simulink model "SIR_Temp2"  (Simulink 7.7)
settings: Solver=ode45  StartTime=0.0  StopTime=inf  MaxStep=.02  RelTol=1e-6  AbsTol=1e-4
InitFcn:
  | Initialization
values from neighbouring files (symbols this model uses):
  g = 9.81    [Initialization.m]
  lenLink1 = 0.5    [Initialization.m]
  lenLink2 = 0.5    [Initialization.m]
  mLink1 = 1    [Initialization.m]
  mLink2 = 1    [Initialization.m]
  mPin1 = 0.5    [Initialization.m]
  mPin2 = 0.5    [Initialization.m]
  rPin1 = 0.025    [Initialization.m]
libraries: mblibv1 x53, simulink x2, vrlib x1
settings Model: Creator=root  LastModifiedBy=root
settings SolverCC: AlgebraicLoopSolver=LineSearch

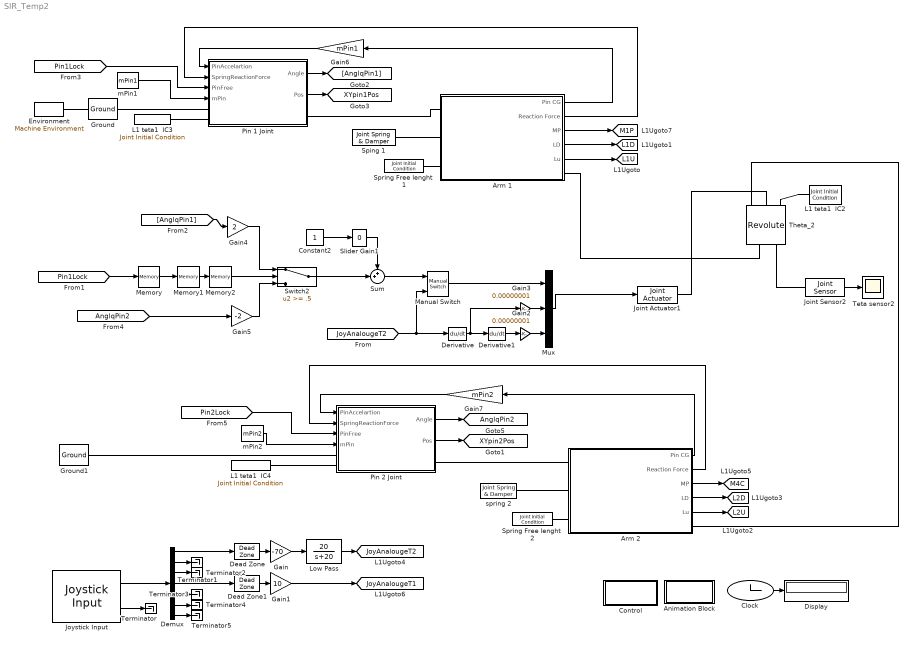
== system SIR_Temp2 ==
  Animation Block : Subsystem
  Arm 1 : Subsystem
  Arm 2 : Subsystem
  Clock : Clock
      settings: Decimation=100
  Constant2 : Constant
  Control : Subsystem
  Dead Zone : DeadZone  LowerValue=-0.1  UpperValue=0.1  SaturateOnIntegerOverflow=on
  Dead Zone1 : DeadZone  LowerValue=-0.1  UpperValue=0.1  SaturateOnIntegerOverflow=on
  Demux : Demux  Outputs=7
  Derivative : Derivative
  Derivative1 : Derivative
  Display : Display
      settings: Decimation=100
  Environment : mblibv1/Bodies/Machine Environment  SystemSampleTime=-1  PortType=env  PhysicalDomain=Mechanical  DialogTemplateClass=MECH.MachineEnvironment  SyncWhenCopied=off  Gravity=[0 -g 0]  GravityUnits=m/s^2  GravityAsSignal=off  Dimensionality=3D Only  AnalysisType=Forward dynamics  LinearAssemblyTolerance=1e-3  LinearAssemblyToleranceUnits=m  AngularAssemblyTolerance=1e-3  AngularAssemblyToleranceUnits=rad  ConstraintSolverType=Stabilizing  ConstraintRelTolerance=1e-4  ConstraintAbsTolerance=1e-4  UseRobustSingularityHandling=off  RedundancyAnalysisToleranceType=Automatically select tolerance  RedundancyAnalysisTolerance=1e-14  StatePerturbationType=Fixed  PerturbationSize=1e-5  VisualizeMachine=on  BodyVisualizationType=Use model default body geometries  BodyColorSelMode=Use model default  DefaultBodyColor=[1 0 0]
  Gain : Gain  Gain=-70
  Gain1 : Gain  Gain=10
  Gain2 : Gain  Gain=0.00000001
  Gain3 : Gain  Gain=0.00000001
  Gain4 : Gain  Gain=2
  Gain5 : Gain  Gain=-2
  Gain6 : Gain  Gain=mPin1
  Gain7 : Gain  Gain=mPin2
  Ground : mblibv1/Bodies/Ground  SystemSampleTime=-1  UpdateFromCAD=off  LeftPortType=env  RightPortType=workingframe  PhysicalDomain=Mechanical  DialogClass=GroundBlock  CoordPosition=[0 0 0]  CoordPositionUnits=m  StateVectorMgrId=1  MachineId=[2 0]  ShowEnvPort=on
  Ground1 : mblibv1/Bodies/Ground  SystemSampleTime=-1  UpdateFromCAD=off  LeftPortType=env  RightPortType=workingframe  PhysicalDomain=Mechanical  DialogClass=GroundBlock  CoordPosition=[0 0 0]  CoordPositionUnits=m  StateVectorMgrId=-1  MachineId=[0 0]  ShowEnvPort=off
  Joint Actuator1 : mblibv1/Sensors &  Actuators/Joint Actuator  SystemSampleTime=-1  UpdateFromCAD=off  PhysicalDomain=Mechanical  PortType=blob  ActuationStyle=Motion  AngleUnits=deg  ArcVelocityUnits=deg/s  ArcAccelerationUnits=deg/s^2  CoordPositionUnits=m  VelocityUnits=m/s  AccelerationUnits=m/s^2  ForceUnits=N  TorqueUnits=N*m  ActiveIO=on  Width=3  DialogClass=MechanicalActuatorBlock  Primitive=R1  ReferenceFrame=Absolute (World)
  Joint Sensor2 : mblibv1/Sensors &  Actuators/Joint Sensor  SystemSampleTime=-1  UpdateFromCAD=off  PhysicalDomain=Mechanical  PortType=blob  Muxed=off  Pose=off  Angle=off  AngleUnits=deg  ArcVelocity=off  ArcVelocityUnits=deg/s  ArcAcceleration=off  ArcAccelerationUnits=deg/s^2  CoordPosition=on  CoordPositionUnits=m  Velocity=off  VelocityUnits=m/s  Acceleration=off  AccelerationUnits=m/s^2  Quaternion=on  QuaternionDT=off  QuaternionDDT=off  QuaternionUnits=off  OutputVector=[1]  ActiveIO=on  Width=3  DialogClass=MechanicalSensorBlock  Primitive=R1  Force=off  ForceUnits=N  Torque=off  TorqueUnits=N*m  ReferenceFrame=Absolute (World)  ReactionSensedSide=Base  ReactionReferenceFrame=Absolute (World)  ReactionForce=off  ReactionForceUnits=N  ReactionMoment=on  ReactionMomentUnits=N*m
  Joystick Input : vrlib/Joystick Input  joyid=1  adjustports=on  forcefeed=off
  L1 teta1  IC2 : mblibv1/Sensors &  Actuators/Joint Initial Condition  SystemSampleTime=-1  UpdateFromCAD=off  LeftPortType=blob  RightPortType=blob  PhysicalDomain=mechanical  DialogClass=InitialConditionBlock  InitialConditions=P1$false$-0.10$m$deg$0$m/s$deg/s#P2$false$0$m$deg$2$m/s$deg/s#P3$false$0$m$deg$0$m/s$deg/s#R1$false$-50$m$deg$0$m/s$deg/s#R2$false$0$m$deg$0$m/s$deg/s#R3$false$0$m$deg$0$m/s$deg/s#S$false$0$m$deg$0$m/s$deg/s  P1PIC=0  P1VIC=0  P2PIC=0  P2VIC=0  P3PIC=0  P3VIC=0  R1PIC=0  R1VIC=0  R2PIC=0  R2VIC=0  R3PIC=0  R3VIC=0  SPIC=0  SVIC=0
  L1 teta1  IC3 : mblibv1/Sensors &  Actuators/Joint Initial Condition  SystemSampleTime=-1  UpdateFromCAD=off  LeftPortType=blob  RightPortType=blob  PhysicalDomain=mechanical  DialogClass=InitialConditionBlock  InitialConditions=P1$false$-0.10$m$deg$0$m/s$deg/s#P2$false$0$m$deg$2$m/s$deg/s#P3$false$0$m$deg$0$m/s$deg/s#R1$true$-60$m$deg$0$m/s$deg/s#R2$false$0$m$deg$0$m/s$deg/s#R3$false$0$m$deg$0$m/s$deg/s#S$false$0$m$deg$0$m/s$deg/s  P1PIC=0  P1VIC=0  P2PIC=0  P2VIC=0  P3PIC=0  P3VIC=0  R1PIC=-60  R1VIC=0  R2PIC=0  R2VIC=0  R3PIC=0  R3VIC=0  SPIC=0  SVIC=0
  L1 teta1  IC4 : mblibv1/Sensors &  Actuators/Joint Initial Condition  SystemSampleTime=-1  UpdateFromCAD=off  LeftPortType=blob  RightPortType=blob  PhysicalDomain=mechanical  DialogClass=InitialConditionBlock  InitialConditions=P1$false$-0.10$m$deg$0$m/s$deg/s#P2$false$0$m$deg$2$m/s$deg/s#P3$false$0$m$deg$0$m/s$deg/s#R1$false$-65$m$deg$0$m/s$deg/s#R2$false$0$m$deg$0$m/s$deg/s#R3$false$0$m$deg$0$m/s$deg/s#S$false$0$m$deg$0$m/s$deg/s  P1PIC=0  P1VIC=0  P2PIC=0  P2VIC=0  P3PIC=0  P3VIC=0  R1PIC=0  R1VIC=0  R2PIC=0  R2VIC=0  R3PIC=0  R3VIC=0  SPIC=0  SVIC=0
  Low Pass : TransferFcn  Numerator=[20]  Denominator=[1 20]
  Manual Switch : simulink/Signal Routing/Manual Switch  SystemSampleTime=-1  sw=1  action=0  varsize=off
  Memory : Memory
  Memory1 : Memory
  Memory2 : Memory
  Mux : Mux  Inputs=3
  Pin 1 Joint : Subsystem
  Pin 2 Joint : Subsystem
  Slider Gain1 : simulink/Math Operations/Slider Gain  SystemSampleTime=-1  low=-100  gain=0  high=100
  Sping 1 : mblibv1/Force  Elements/Joint Spring & Damper  SystemSampleTime=-1  UpdateFromCAD=off  DialogClass=JointSpringDamper  JFEParameters=P1$true$sK1$0$sFl1$m$m/s$N$deg$deg/s$N*m#P2$false$0$0$0$m$m/s$N$deg$deg/s$N*m#P3$false$0$0$0$m$m/s$N$deg$deg/s$N*m#R1$false$0$.02$0$m$m/s$N$deg$deg/s$N*m#R2$false$0$0$0$m$m/s$N$deg$deg/s$N*m#R3$false$0$0$0$m$m/s$N$deg$deg/s$N*m#S$false$0$0$0$m$m/s$N$deg$deg/s$N*m
  Spring Free lenght  1 : mblibv1/Sensors &  Actuators/Joint Initial Condition  SystemSampleTime=-1  UpdateFromCAD=off  LeftPortType=blob  RightPortType=blob  PhysicalDomain=mechanical  DialogClass=InitialConditionBlock  InitialConditions=P1$true$sFl1$m$deg$0$m/s$deg/s#P2$false$0$m$deg$2$m/s$deg/s#P3$false$0$m$deg$0$m/s$deg/s#R1$false$-65$m$deg$0$m/s$deg/s#R2$false$0$m$deg$0$m/s$deg/s#R3$false$0$m$deg$0$m/s$deg/s#S$false$0$m$deg$0$m/s$deg/s  P1PIC=sFl1  P1VIC=0  P2PIC=0  P2VIC=0  P3PIC=0  P3VIC=0  R1PIC=0  R1VIC=0  R2PIC=0  R2VIC=0  R3PIC=0  R3VIC=0  SPIC=0  SVIC=0
  Spring Free lenght  2 : mblibv1/Sensors &  Actuators/Joint Initial Condition  SystemSampleTime=-1  UpdateFromCAD=off  LeftPortType=blob  RightPortType=blob  PhysicalDomain=mechanical  DialogClass=InitialConditionBlock  InitialConditions=P1$true$sFl1$m$deg$0$m/s$deg/s#P2$false$0$m$deg$2$m/s$deg/s#P3$false$0$m$deg$0$m/s$deg/s#R1$false$-65$m$deg$0$m/s$deg/s#R2$false$0$m$deg$0$m/s$deg/s#R3$false$0$m$deg$0$m/s$deg/s#S$false$0$m$deg$0$m/s$deg/s  P1PIC=sFl1  P1VIC=0  P2PIC=0  P2VIC=0  P3PIC=0  P3VIC=0  R1PIC=0  R1VIC=0  R2PIC=0  R2VIC=0  R3PIC=0  R3VIC=0  SPIC=0  SVIC=0
  Sum : Sum  Inputs=++|
  Switch2 : Switch  Threshold=.5
  Terminator{,1..5} (6 alike) : Terminator
  Teta sensor2 : Scope
      settings: TimeRange=45  YMin=-10  YMax=10  SaveName=ScopeData6
  Theta_2 : mblibv1/Joints/Revolute  PhysicalDomain=mechanical  SubClassName=Unknown  LeftPortType=blob  RightPortType=blob  LConnTagsString=__newl0|SA1|SA2  RConnTagsString=__newr0|SA1  UpdateFromCAD=off  NumSAPorts=3  CutJoint=off  MarkAsCut=off  Primitives=prismatic  PrimitiveProps=R1$Follower$[0 0 1]$revolute  DialogClass=JointBlock  R1Axis=[0 0 1]
  mPin1 : Constant  Value=mPin1
  mPin2 : Constant  Value=mPin2
  spring 2 : mblibv1/Force  Elements/Joint Spring & Damper  SystemSampleTime=-1  UpdateFromCAD=off  DialogClass=JointSpringDamper  JFEParameters=P1$true$sK2$0$sFl2$m$m/s$N$deg$deg/s$N*m#P2$false$0$0$0$m$m/s$N$deg$deg/s$N*m#P3$false$0$0$0$m$m/s$N$deg$deg/s$N*m#R1$false$0$0$0$m$m/s$N$deg$deg/s$N*m#R2$false$0$0$0$m$m/s$N$deg$deg/s$N*m#R3$false$0$0$0$m$m/s$N$deg$deg/s$N*m#S$false$0$0$0$m$m/s$N$deg$deg/s$N*m
  tag scope: AnglqPin2=global, JoyAnalougeT1=global, JoyAnalougeT2=global, L1D=global, L1U=global, L2D=global, L2U=global, M1P=global, M4C=global, XYpin1Pos=global, XYpin2Pos=global
  wires:
  Clock/1 -> Display/1
  Joystick Input/1 -> Demux/1
  Joystick Input/2 -> Terminator/1
  Demux/3 -> Terminator2/1
  Demux/4 -> Dead Zone1/1
  Demux/5 -> Terminator3/1
  Demux/6 -> Terminator4/1
  Demux/7 -> Terminator5/1
  Dead Zone/1 -> Gain/1
  Gain/1 -> Low Pass/1
  Dead Zone1/1 -> Gain1/1
  Gain1/1 -> [JoyAnalougeT1]
  Demux/1 -> Dead Zone/1
  Demux/2 -> Terminator1/1
  Derivative/1 -> Derivative1/1, Gain3/1
  Derivative1/1 -> Gain2/1
  Low Pass/1 -> [JoyAnalougeT2]
  Joint Sensor2/1 -> Teta sensor2/1
  Gain2/1 -> Mux/3
  Gain3/1 -> Mux/2
  Arm 1/1(Pin CG) -> Gain6/1
  Gain6/1 -> Pin 1 Joint/1(PinAccelartion)
  [Pin1Lock] -> Memory/1
  mPin1/1 -> Pin 1 Joint/4(mPin)
  Pin 1 Joint/1(Angle) -> [AnglqPin1]
  Arm 1/2(Reaction Force) -> Pin 1 Joint/2(SpringReactionForce)
  Arm 1/3(MP) -> [M1P]
  Arm 1/4(LD) -> [L1D]
  Arm 1/5(Lu) -> [L1U]
  [AnglqPin1] -> Gain4/1
  Arm 2/3(MP) -> [M4C]
  Arm 2/1(Pin CG) -> Gain7/1
  mPin2/1 -> Pin 2 Joint/4(mPin)
  Constant2/1 -> Slider Gain1/1
  Slider Gain1/1 -> Sum/1
  Pin 2 Joint/1(Angle) -> [AnglqPin2]
  Pin 1 Joint/2(Pos) -> [XYpin1Pos]
  Pin 2 Joint/2(Pos) -> [XYpin2Pos]
  Memory/1 -> Memory1/1
  Memory1/1 -> Memory2/1
  Memory2/1 -> Switch2/2
  Arm 2/4(LD) -> [L2D]
  Arm 2/5(Lu) -> [L2U]
  [Pin1Lock] -> Pin 1 Joint/3(PinFree)
  Gain7/1 -> Pin 2 Joint/1(PinAccelartion)
  Arm 2/2(Reaction Force) -> Pin 2 Joint/2(SpringReactionForce)
  [Pin2Lock] -> Pin 2 Joint/3(PinFree)
  Gain4/1 -> Switch2/1
  [AnglqPin2] -> Gain5/1
  Gain5/1 -> Switch2/3
  Switch2/1 -> Sum/2
  Mux/1 -> Joint Actuator1/1
  Sum/1 -> Manual Switch/1
  Manual Switch/1 -> Mux/1
  [JoyAnalougeT2] -> Derivative/1, Manual Switch/2
  connections:
  Ground/LConn1 -- Environment/RConn1
  Joint Sensor2/LConn1 -- Theta_2/RConn2
  L1 teta1  IC2/RConn1 -- Theta_2/LConn3
  Ground/RConn1 -- Pin 1 Joint/LConn1
  Joint Actuator1/RConn1 -- Theta_2/LConn2
  Pin 1 Joint/RConn1 -- Arm 1/LConn1
  L1 teta1  IC3/RConn1 -- Pin 1 Joint/LConn2
  Sping 1/LConn1 -- Arm 1/LConn2
  Spring Free lenght  1/RConn1 -- Arm 1/LConn3
  spring 2/LConn1 -- Arm 2/LConn2
  Arm 2/LConn3 -- Spring Free lenght  2/RConn1
  Pin 2 Joint/LConn1 -- Ground1/RConn1
  L1 teta1  IC4/RConn1 -- Pin 2 Joint/LConn2
  Arm 2/LConn1 -- Pin 2 Joint/RConn1
  Theta_2/RConn1 -- Arm 1/RConn1
  Theta_2/LConn1 -- Arm 2/RConn1

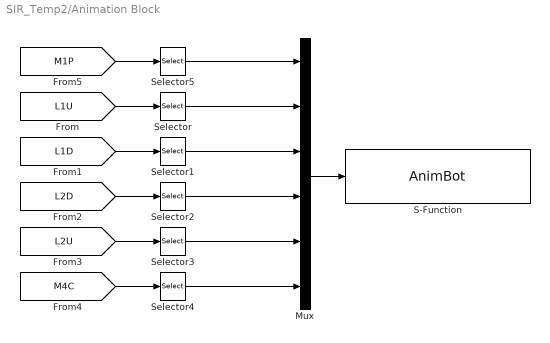
== system SIR_Temp2/Animation Block ==
  Mux : Mux  Inputs=6
  S-Function : S-Function  FunctionName=AnimBot  Parameters=0.001  EnableBusSupport=off
  Selector{,1..5} (6 alike) : Selector  InputPortWidth=3  IndexOptions=Index vector (dialog)  Indices=[1 2]  OutputSizes=1
  wires:
  Mux/1 -> S-Function/1
  [M4C] -> Selector4/1
  [L2U] -> Selector3/1
  [L2D] -> Selector2/1
  [L1D] -> Selector1/1
  [L1U] -> Selector/1
  [M1P] -> Selector5/1
  Selector5/1 -> Mux/1
  Selector/1 -> Mux/2
  Selector1/1 -> Mux/3
  Selector2/1 -> Mux/4
  Selector3/1 -> Mux/5
  Selector4/1 -> Mux/6

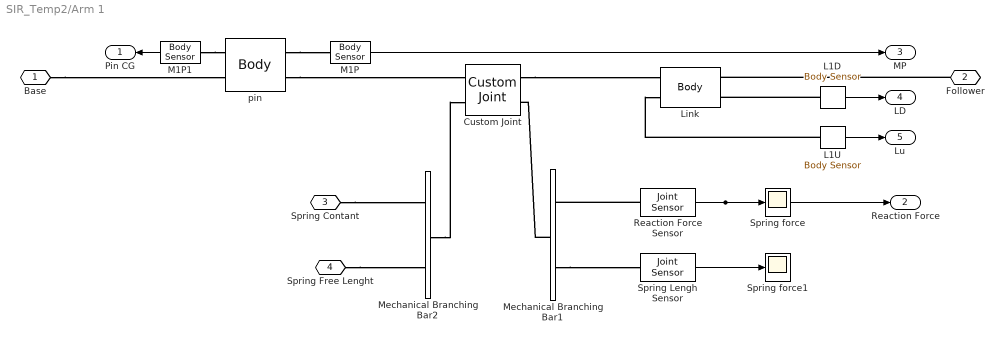
== system SIR_Temp2/Arm 1 ==
  Custom Joint : mblibv1/Joints/Custom Joint  PhysicalDomain=mechanical  SubClassName=custom_joint  LeftPortType=blob  RightPortType=blob  LConnTagsString=__newl0|SA1  RConnTagsString=__newr0|SA1  UpdateFromCAD=off  NumSAPorts=2  CutJoint=off  MarkAsCut=off  Primitives=prismatic  PrimitiveProps=P1$World$[0 1 0]$Prismatic  DialogClass=JointBlock  R1Axis=[]  R2Axis=[]  R3Axis=[]  P1Axis=[0 1 0]  P2Axis=[]  P3Axis=[]  SAxis=[]
  L1D : mblibv1/Sensors &  Actuators/Body Sensor  SystemSampleTime=-1  UpdateFromCAD=off  PhysicalDomain=Mechanical  PortType=blob  Muxed=on  Pose=off  Angle=on  AngleUnits=deg  ArcVelocity=off  ArcVelocityUnits=deg/s  ArcAcceleration=off  ArcAccelerationUnits=deg/s^2  CoordPosition=on  CoordPositionUnits=m  Velocity=off  VelocityUnits=m/s  Acceleration=off  AccelerationUnits=m/s^2  Quaternion=on  QuaternionDT=off  QuaternionDDT=off  QuaternionUnits=off  OutputVector=[1]  ActiveIO=on  Width=3  DialogClass=MechanicalSensorBlock  ReferenceFrame=Absolute (World)
  L1U : mblibv1/Sensors &  Actuators/Body Sensor  SystemSampleTime=-1  UpdateFromCAD=off  PhysicalDomain=Mechanical  PortType=blob  Muxed=on  Pose=off  Angle=on  AngleUnits=deg  ArcVelocity=off  ArcVelocityUnits=deg/s  ArcAcceleration=off  ArcAccelerationUnits=deg/s^2  CoordPosition=on  CoordPositionUnits=m  Velocity=off  VelocityUnits=m/s  Acceleration=off  AccelerationUnits=m/s^2  Quaternion=on  QuaternionDT=off  QuaternionDDT=off  QuaternionUnits=off  OutputVector=[1]  ActiveIO=on  Width=3  DialogClass=MechanicalSensorBlock  ReferenceFrame=Absolute (World)
  Link : mblibv1/Bodies/Body  PhysicalDomain=mechanical  SubClassName=Unknown  LeftPortType=workingframe  RightPortType=workingframe  LConnTagsString=CS1|CS3  RConnTagsString=CS2|CS4  UpdateFromCAD=off  DialogClass=MechanicalBodyBlock  Mass=mLink1  MassUnits=kg  InertiaUnits=kg*m^2  Inertia=mLink1/12*[lenLink1 0 0; 0 0 0; 0 0 lenLink1]  Shape=Cylinder  ShapeDims=[1 1]  ShapeUnits=m  ShapeUse=false  Density=1  DensityUnits=kg/m^3  DensityUse=false  GraphicsMode=MACHINE_DEFAULT  BodyColorSelMode=MACHINE_DEFAULT  BodyColor=[1 0 0]  AttachedToCS=CG  CG=Left$CG$[0 -0.25 0]$CS1$CS1$m$[0 0 0]$Euler X-Y-Z$deg$WORLD$false$none  WorkingFrames=Left$CS1$[0 0 0]$Adjoining$Adjoining$m$[0 0 0]$Euler X-Y-Z$deg$WORLD$true$none#Left$CS3$[0 0 0]$CS1$CS1$m$[0 0 0]$Euler X-Y-Z$deg$WORLD$true$none#Right$CS2$[0 -0.5 0]$CS1$CS1$m$[0 0 0]$Euler X-Y-Z$deg$WORLD$true$none#Right$CS4$[0 -0.5 0]$CS1$CS1$m$[0 0 0]$Euler X-Y-Z$deg$WORLD$true$none  CGPos=[0 -0.25 0]  CGRot=[0 0 0]  CS0Pos=[]  CS0Rot=[]  CS1Pos=[0 0 0]  CS1Rot=[0 0 0]  CS2Pos=[0 -0.5 0]  CS2Rot=[0 0 0]  CS3Pos=[0 0 0]  CS3Rot=[0 0 0]  CS4Pos=[0 -0.5 0]  CS4Rot=[0 0 0]  CS5Pos=[]  CS5Rot=[]  CS6Pos=[]  CS6Rot=[]  CS7Pos=[]  CS7Rot=[]  CS8Pos=[]  CS8Rot=[]  CS9Pos=[]  CS9Rot=[]  CS10Pos=[]  CS10Rot=[]  CS11Pos=[]  CS11Rot=[]  CS12Pos=[]  CS12Rot=[]  CS13Pos=[]  CS13Rot=[]  CS14Pos=[]  CS14Rot=[]  CS15Pos=[]  CS15Rot=[]  CS16Pos=[]  CS16Rot=[]  CS17Pos=[]  CS17Rot=[]  CS18Pos=[]  CS18Rot=[]  CS19Pos=[]  CS19Rot=[]  CS20Pos=[]  CS20Rot=[]
  M1P : mblibv1/Sensors &  Actuators/Body Sensor  SystemSampleTime=-1  UpdateFromCAD=off  PhysicalDomain=Mechanical  PortType=blob  Muxed=on  Pose=off  Angle=on  AngleUnits=deg  ArcVelocity=off  ArcVelocityUnits=deg/s  ArcAcceleration=off  ArcAccelerationUnits=deg/s^2  CoordPosition=on  CoordPositionUnits=m  Velocity=off  VelocityUnits=m/s  Acceleration=off  AccelerationUnits=m/s^2  Quaternion=on  QuaternionDT=off  QuaternionDDT=off  QuaternionUnits=off  OutputVector=[1]  ActiveIO=on  Width=3  DialogClass=MechanicalSensorBlock  ReferenceFrame=Absolute (World)
  M1P1 : mblibv1/Sensors &  Actuators/Body Sensor  SystemSampleTime=-1  UpdateFromCAD=off  PhysicalDomain=Mechanical  PortType=blob  Muxed=on  Pose=off  Angle=on  AngleUnits=deg  ArcVelocity=off  ArcVelocityUnits=deg/s  ArcAcceleration=off  ArcAccelerationUnits=deg/s^2  CoordPosition=off  CoordPositionUnits=m  Velocity=off  VelocityUnits=m/s  Acceleration=on  AccelerationUnits=m/s^2  Quaternion=on  QuaternionDT=off  QuaternionDDT=off  QuaternionUnits=off  OutputVector=[1]  ActiveIO=on  Width=3  DialogClass=MechanicalSensorBlock  ReferenceFrame=Absolute (World)
  Mechanical Branching Bar1 : mblibv1/Utilities/Mechanical Branching Bar  PhysicalDomain=mechanical  SubClassName=Unknown  LeftPortType=blob  RightPortType=blob  LConnTagsString=_newl0  RConnTagsString=__newr0|SA2  UpdateFromCAD=off  DialogClass=MechanicalBranchingBarBlock  NumSAPorts=2
  Mechanical Branching Bar2 : mblibv1/Utilities/Mechanical Branching Bar  PhysicalDomain=mechanical  SubClassName=Unknown  LeftPortType=blob  RightPortType=blob  LConnTagsString=_newl0  RConnTagsString=__newr0|SA2  UpdateFromCAD=off  DialogClass=MechanicalBranchingBarBlock  NumSAPorts=2
  "Reaction Force Sensor " : mblibv1/Sensors &  Actuators/Joint Sensor  SystemSampleTime=-1  UpdateFromCAD=off  PhysicalDomain=Mechanical  PortType=blob  Muxed=off  Pose=off  Angle=on  AngleUnits=deg  ArcVelocity=off  ArcVelocityUnits=deg/s  ArcAcceleration=off  ArcAccelerationUnits=deg/s^2  CoordPosition=off  CoordPositionUnits=m  Velocity=off  VelocityUnits=m/s  Acceleration=off  AccelerationUnits=m/s^2  Quaternion=on  QuaternionDT=off  QuaternionDDT=off  QuaternionUnits=off  OutputVector=[1]  ActiveIO=on  Width=3  DialogClass=MechanicalSensorBlock  Primitive=P1  Force=off  ForceUnits=N  Torque=off  TorqueUnits=N*m  ReferenceFrame=Absolute (World)  ReactionSensedSide=Base  ReactionReferenceFrame=Absolute (World)  ReactionForce=on  ReactionForceUnits=N  ReactionMoment=off  ReactionMomentUnits=N*m
  Spring Lengh Sensor : mblibv1/Sensors &  Actuators/Joint Sensor  SystemSampleTime=-1  UpdateFromCAD=off  PhysicalDomain=Mechanical  PortType=blob  Muxed=off  Pose=off  Angle=on  AngleUnits=deg  ArcVelocity=off  ArcVelocityUnits=deg/s  ArcAcceleration=off  ArcAccelerationUnits=deg/s^2  CoordPosition=off  CoordPositionUnits=m  Velocity=off  VelocityUnits=m/s  Acceleration=off  AccelerationUnits=m/s^2  Quaternion=on  QuaternionDT=off  QuaternionDDT=off  QuaternionUnits=off  OutputVector=[1]  ActiveIO=on  Width=3  DialogClass=MechanicalSensorBlock  Primitive=P1  Force=off  ForceUnits=N  Torque=off  TorqueUnits=N*m  ReferenceFrame=Absolute (World)  ReactionSensedSide=Base  ReactionReferenceFrame=Absolute (World)  ReactionForce=on  ReactionForceUnits=N  ReactionMoment=off  ReactionMomentUnits=N*m
  Spring force : Scope
      settings: TimeRange=0.45  YMin=-10  YMax=1  SaveName=ScopeData22
  Spring force1 : Scope
      settings: TimeRange=0.45  YMin=-10  YMax=1  SaveName=ScopeData8
  pin : mblibv1/Bodies/Body  PhysicalDomain=mechanical  SubClassName=Unknown  LeftPortType=workingframe  RightPortType=workingframe  LConnTagsString=CG|CS3  RConnTagsString=CS2|CS4  UpdateFromCAD=off  DialogClass=MechanicalBodyBlock  Mass=mPin1  MassUnits=kg  InertiaUnits=kg*m^2  Inertia=2/5*mPin1*(rPin1)^2*[1 0 0; 0 1 0; 0 0 1]  Shape=Cylinder  ShapeDims=[1 1]  ShapeUnits=m  ShapeUse=false  Density=1  DensityUnits=kg/m^3  DensityUse=false  GraphicsMode=MACHINE_DEFAULT  BodyColorSelMode=MACHINE_DEFAULT  BodyColor=[1 0 0]  AttachedToCS=CG  CG=Left$CG$[0 -0.025 0]$CS3$CS3$m$[0 0 0]$Euler X-Y-Z$deg$WORLD$true$none  WorkingFrames=Left$CS3$[0 0 0]$Adjoining$Adjoining$m$[0 0 0]$Euler X-Y-Z$deg$WORLD$true$none#Right$CS2$[0 -.025 0]$CS3$CS3$m$[0 0 0]$Euler X-Y-Z$deg$WORLD$true$none#Right$CS4$[0 -.05 0]$CS3$CS3$m$[0 0 0]$Euler X-Y-Z$deg$WORLD$true$none  CGPos=[0 -0.025 0]  CGRot=[0 0 0]  CS0Pos=[]  CS0Rot=[]  CS1Pos=[]  CS1Rot=[]  CS2Pos=[0 -.025 0]  CS2Rot=[0 0 0]  CS3Pos=[0 0 0]  CS3Rot=[0 0 0]  CS4Pos=[0 -.05 0]  CS4Rot=[0 0 0]  CS5Pos=[]  CS5Rot=[]  CS6Pos=[]  CS6Rot=[]  CS7Pos=[]  CS7Rot=[]  CS8Pos=[]  CS8Rot=[]  CS9Pos=[]  CS9Rot=[]  CS10Pos=[]  CS10Rot=[]  CS11Pos=[]  CS11Rot=[]  CS12Pos=[]  CS12Rot=[]  CS13Pos=[]  CS13Rot=[]  CS14Pos=[]  CS14Rot=[]  CS15Pos=[]  CS15Rot=[]  CS16Pos=[]  CS16Rot=[]  CS17Pos=[]  CS17Rot=[]  CS18Pos=[]  CS18Rot=[]  CS19Pos=[]  CS19Rot=[]  CS20Pos=[]  CS20Rot=[]
  Base : PMIOPort  Port=1  Side=Left
  Follower : PMIOPort  Port=2  Side=Right
  Spring Contant : PMIOPort  Port=3  Side=Left
  Spring Free Lenght : PMIOPort  Port=4  Side=Left
  Pin CG : Outport
  Reaction Force : Outport  Port=2
  MP : Outport  Port=3
  LD : Outport  Port=4
  Lu : Outport  Port=5
  wires:
  L1U/1 -> Lu/1
  L1D/1 -> LD/1
  M1P1/1 -> Pin CG/1
  "Reaction Force Sensor "/1 -> Reaction Force/1, Spring force/1
  Spring Lengh Sensor/1 -> Spring force1/1
  M1P/1 -> MP/1
  connections:
  pin/RConn2 -- Custom Joint/LConn1
  Mechanical Branching Bar2/LConn1 -- Custom Joint/LConn2
  Mechanical Branching Bar1/LConn1 -- Custom Joint/RConn2
  L1D/LConn1 -- Link/RConn2
  L1U/LConn1 -- Link/LConn2
  pin/RConn1 -- M1P/LConn1
  M1P1/LConn1 -- pin/LConn1
  "Reaction Force Sensor "/LConn1 -- Mechanical Branching Bar1/RConn1
  Base/RConn1 -- pin/LConn2
  Follower/RConn1 -- Link/RConn1
  Custom Joint/RConn1 -- Link/LConn1
  Mechanical Branching Bar1/RConn2 -- Spring Lengh Sensor/LConn1
  Spring Contant/RConn1 -- Mechanical Branching Bar2/RConn1
  Spring Free Lenght/RConn1 -- Mechanical Branching Bar2/RConn2

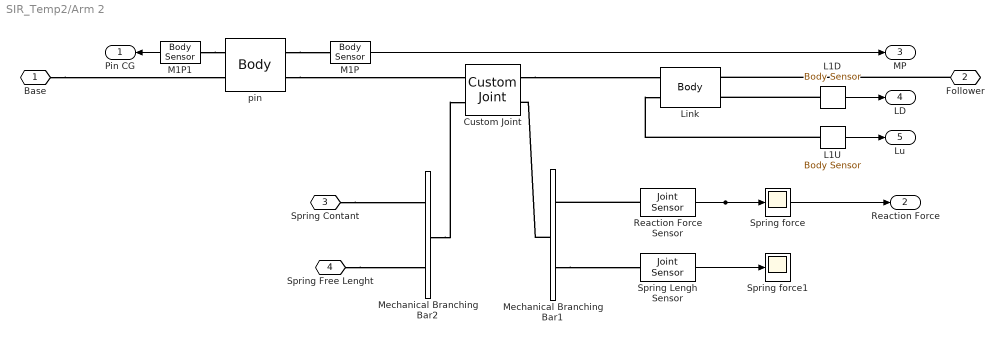
== system SIR_Temp2/Arm 2 ==
  Custom Joint : mblibv1/Joints/Custom Joint  PhysicalDomain=mechanical  SubClassName=custom_joint  LeftPortType=blob  RightPortType=blob  LConnTagsString=__newl0|SA1  RConnTagsString=__newr0|SA1  UpdateFromCAD=off  NumSAPorts=2  CutJoint=off  MarkAsCut=off  Primitives=prismatic  PrimitiveProps=P1$World$[0 1 0]$Prismatic  DialogClass=JointBlock  R1Axis=[]  R2Axis=[]  R3Axis=[]  P1Axis=[0 1 0]  P2Axis=[]  P3Axis=[]  SAxis=[]
  L1D : mblibv1/Sensors &  Actuators/Body Sensor  SystemSampleTime=-1  UpdateFromCAD=off  PhysicalDomain=Mechanical  PortType=blob  Muxed=on  Pose=off  Angle=on  AngleUnits=deg  ArcVelocity=off  ArcVelocityUnits=deg/s  ArcAcceleration=off  ArcAccelerationUnits=deg/s^2  CoordPosition=on  CoordPositionUnits=m  Velocity=off  VelocityUnits=m/s  Acceleration=off  AccelerationUnits=m/s^2  Quaternion=on  QuaternionDT=off  QuaternionDDT=off  QuaternionUnits=off  OutputVector=[1]  ActiveIO=on  Width=3  DialogClass=MechanicalSensorBlock  ReferenceFrame=Absolute (World)
  L1U : mblibv1/Sensors &  Actuators/Body Sensor  SystemSampleTime=-1  UpdateFromCAD=off  PhysicalDomain=Mechanical  PortType=blob  Muxed=on  Pose=off  Angle=on  AngleUnits=deg  ArcVelocity=off  ArcVelocityUnits=deg/s  ArcAcceleration=off  ArcAccelerationUnits=deg/s^2  CoordPosition=on  CoordPositionUnits=m  Velocity=off  VelocityUnits=m/s  Acceleration=off  AccelerationUnits=m/s^2  Quaternion=on  QuaternionDT=off  QuaternionDDT=off  QuaternionUnits=off  OutputVector=[1]  ActiveIO=on  Width=3  DialogClass=MechanicalSensorBlock  ReferenceFrame=Absolute (World)
  Link : mblibv1/Bodies/Body  PhysicalDomain=mechanical  SubClassName=Unknown  LeftPortType=workingframe  RightPortType=workingframe  LConnTagsString=CS1|CS3  RConnTagsString=CS2|CS4  UpdateFromCAD=off  DialogClass=MechanicalBodyBlock  Mass=mLink2  MassUnits=kg  InertiaUnits=kg*m^2  Inertia=mLink2/12*[lenLink2 0 0; 0 0 0; 0 0 lenLink2]  Shape=Cylinder  ShapeDims=[1 1]  ShapeUnits=m  ShapeUse=false  Density=1  DensityUnits=kg/m^3  DensityUse=false  GraphicsMode=MACHINE_DEFAULT  BodyColorSelMode=MACHINE_DEFAULT  BodyColor=[1 0 0]  AttachedToCS=CG  CG=Left$CG$[0 -0.25 0]$CS1$CS1$m$[0 0 0]$Euler X-Y-Z$deg$WORLD$false$none  WorkingFrames=Left$CS1$[0 0 0]$Adjoining$Adjoining$m$[0 0 0]$Euler X-Y-Z$deg$WORLD$true$none#Left$CS3$[0 0 0]$CS1$CS1$m$[0 0 0]$Euler X-Y-Z$deg$WORLD$true$none#Right$CS2$[0 -0.5 0]$CS1$CS1$m$[0 0 0]$Euler X-Y-Z$deg$WORLD$true$none#Right$CS4$[0 -0.5 0]$CS1$CS1$m$[0 0 0]$Euler X-Y-Z$deg$WORLD$true$none  CGPos=[0 -0.25 0]  CGRot=[0 0 0]  CS0Pos=[]  CS0Rot=[]  CS1Pos=[0 0 0]  CS1Rot=[0 0 0]  CS2Pos=[0 -0.5 0]  CS2Rot=[0 0 0]  CS3Pos=[0 0 0]  CS3Rot=[0 0 0]  CS4Pos=[0 -0.5 0]  CS4Rot=[0 0 0]  CS5Pos=[]  CS5Rot=[]  CS6Pos=[]  CS6Rot=[]  CS7Pos=[]  CS7Rot=[]  CS8Pos=[]  CS8Rot=[]  CS9Pos=[]  CS9Rot=[]  CS10Pos=[]  CS10Rot=[]  CS11Pos=[]  CS11Rot=[]  CS12Pos=[]  CS12Rot=[]  CS13Pos=[]  CS13Rot=[]  CS14Pos=[]  CS14Rot=[]  CS15Pos=[]  CS15Rot=[]  CS16Pos=[]  CS16Rot=[]  CS17Pos=[]  CS17Rot=[]  CS18Pos=[]  CS18Rot=[]  CS19Pos=[]  CS19Rot=[]  CS20Pos=[]  CS20Rot=[]
  M1P : mblibv1/Sensors &  Actuators/Body Sensor  SystemSampleTime=-1  UpdateFromCAD=off  PhysicalDomain=Mechanical  PortType=blob  Muxed=on  Pose=off  Angle=on  AngleUnits=deg  ArcVelocity=off  ArcVelocityUnits=deg/s  ArcAcceleration=off  ArcAccelerationUnits=deg/s^2  CoordPosition=on  CoordPositionUnits=m  Velocity=off  VelocityUnits=m/s  Acceleration=off  AccelerationUnits=m/s^2  Quaternion=on  QuaternionDT=off  QuaternionDDT=off  QuaternionUnits=off  OutputVector=[1]  ActiveIO=on  Width=3  DialogClass=MechanicalSensorBlock  ReferenceFrame=Absolute (World)
  M1P1 : mblibv1/Sensors &  Actuators/Body Sensor  SystemSampleTime=-1  UpdateFromCAD=off  PhysicalDomain=Mechanical  PortType=blob  Muxed=on  Pose=off  Angle=on  AngleUnits=deg  ArcVelocity=off  ArcVelocityUnits=deg/s  ArcAcceleration=off  ArcAccelerationUnits=deg/s^2  CoordPosition=off  CoordPositionUnits=m  Velocity=off  VelocityUnits=m/s  Acceleration=on  AccelerationUnits=m/s^2  Quaternion=on  QuaternionDT=off  QuaternionDDT=off  QuaternionUnits=off  OutputVector=[1]  ActiveIO=on  Width=3  DialogClass=MechanicalSensorBlock  ReferenceFrame=Absolute (World)
  Mechanical Branching Bar1 : mblibv1/Utilities/Mechanical Branching Bar  PhysicalDomain=mechanical  SubClassName=Unknown  LeftPortType=blob  RightPortType=blob  LConnTagsString=_newl0  RConnTagsString=__newr0|SA2  UpdateFromCAD=off  DialogClass=MechanicalBranchingBarBlock  NumSAPorts=2
  Mechanical Branching Bar2 : mblibv1/Utilities/Mechanical Branching Bar  PhysicalDomain=mechanical  SubClassName=Unknown  LeftPortType=blob  RightPortType=blob  LConnTagsString=_newl0  RConnTagsString=__newr0|SA2  UpdateFromCAD=off  DialogClass=MechanicalBranchingBarBlock  NumSAPorts=2
  "Reaction Force Sensor " : mblibv1/Sensors &  Actuators/Joint Sensor  SystemSampleTime=-1  UpdateFromCAD=off  PhysicalDomain=Mechanical  PortType=blob  Muxed=off  Pose=off  Angle=on  AngleUnits=deg  ArcVelocity=off  ArcVelocityUnits=deg/s  ArcAcceleration=off  ArcAccelerationUnits=deg/s^2  CoordPosition=off  CoordPositionUnits=m  Velocity=off  VelocityUnits=m/s  Acceleration=off  AccelerationUnits=m/s^2  Quaternion=on  QuaternionDT=off  QuaternionDDT=off  QuaternionUnits=off  OutputVector=[1]  ActiveIO=on  Width=3  DialogClass=MechanicalSensorBlock  Primitive=P1  Force=off  ForceUnits=N  Torque=off  TorqueUnits=N*m  ReferenceFrame=Absolute (World)  ReactionSensedSide=Base  ReactionReferenceFrame=Absolute (World)  ReactionForce=on  ReactionForceUnits=N  ReactionMoment=off  ReactionMomentUnits=N*m
  Spring Lengh Sensor : mblibv1/Sensors &  Actuators/Joint Sensor  SystemSampleTime=-1  UpdateFromCAD=off  PhysicalDomain=Mechanical  PortType=blob  Muxed=off  Pose=off  Angle=on  AngleUnits=deg  ArcVelocity=off  ArcVelocityUnits=deg/s  ArcAcceleration=off  ArcAccelerationUnits=deg/s^2  CoordPosition=off  CoordPositionUnits=m  Velocity=off  VelocityUnits=m/s  Acceleration=off  AccelerationUnits=m/s^2  Quaternion=on  QuaternionDT=off  QuaternionDDT=off  QuaternionUnits=off  OutputVector=[1]  ActiveIO=on  Width=3  DialogClass=MechanicalSensorBlock  Primitive=P1  Force=off  ForceUnits=N  Torque=off  TorqueUnits=N*m  ReferenceFrame=Absolute (World)  ReactionSensedSide=Base  ReactionReferenceFrame=Absolute (World)  ReactionForce=on  ReactionForceUnits=N  ReactionMoment=off  ReactionMomentUnits=N*m
  Spring force : Scope
      settings: TimeRange=0.45  YMin=-10  YMax=1  SaveName=ScopeData22
  Spring force1 : Scope
      settings: TimeRange=0.45  YMin=-10  YMax=1  SaveName=ScopeData8
  pin : mblibv1/Bodies/Body  PhysicalDomain=mechanical  SubClassName=Unknown  LeftPortType=workingframe  RightPortType=workingframe  LConnTagsString=CG|CS3  RConnTagsString=CS2|CS4  UpdateFromCAD=off  DialogClass=MechanicalBodyBlock  Mass=mPin1  MassUnits=kg  InertiaUnits=kg*m^2  Inertia=2/5*mPin1*(rPin1)^2*[1 0 0; 0 1 0; 0 0 1]  Shape=Cylinder  ShapeDims=[1 1]  ShapeUnits=m  ShapeUse=false  Density=1  DensityUnits=kg/m^3  DensityUse=false  GraphicsMode=MACHINE_DEFAULT  BodyColorSelMode=MACHINE_DEFAULT  BodyColor=[1 0 0]  AttachedToCS=CG  CG=Left$CG$[0 -0.025 0]$CS3$CS3$m$[0 0 0]$Euler X-Y-Z$deg$WORLD$true$none  WorkingFrames=Left$CS3$[0 0 0]$Adjoining$Adjoining$m$[0 0 0]$Euler X-Y-Z$deg$WORLD$true$none#Right$CS2$[0 -.025 0]$CS3$CS3$m$[0 0 0]$Euler X-Y-Z$deg$WORLD$true$none#Right$CS4$[0 -.05 0]$CS3$CS3$m$[0 0 0]$Euler X-Y-Z$deg$WORLD$true$none  CGPos=[0 -0.025 0]  CGRot=[0 0 0]  CS0Pos=[]  CS0Rot=[]  CS1Pos=[]  CS1Rot=[]  CS2Pos=[0 -.025 0]  CS2Rot=[0 0 0]  CS3Pos=[0 0 0]  CS3Rot=[0 0 0]  CS4Pos=[0 -.05 0]  CS4Rot=[0 0 0]  CS5Pos=[]  CS5Rot=[]  CS6Pos=[]  CS6Rot=[]  CS7Pos=[]  CS7Rot=[]  CS8Pos=[]  CS8Rot=[]  CS9Pos=[]  CS9Rot=[]  CS10Pos=[]  CS10Rot=[]  CS11Pos=[]  CS11Rot=[]  CS12Pos=[]  CS12Rot=[]  CS13Pos=[]  CS13Rot=[]  CS14Pos=[]  CS14Rot=[]  CS15Pos=[]  CS15Rot=[]  CS16Pos=[]  CS16Rot=[]  CS17Pos=[]  CS17Rot=[]  CS18Pos=[]  CS18Rot=[]  CS19Pos=[]  CS19Rot=[]  CS20Pos=[]  CS20Rot=[]
  Base : PMIOPort  Port=1  Side=Left
  Follower : PMIOPort  Port=2  Side=Right
  Spring Contant : PMIOPort  Port=3  Side=Left
  Spring Free Lenght : PMIOPort  Port=4  Side=Left
  Pin CG : Outport
  Reaction Force : Outport  Port=2
  MP : Outport  Port=3
  LD : Outport  Port=4
  Lu : Outport  Port=5
  wires:
  L1U/1 -> Lu/1
  L1D/1 -> LD/1
  M1P1/1 -> Pin CG/1
  "Reaction Force Sensor "/1 -> Reaction Force/1, Spring force/1
  Spring Lengh Sensor/1 -> Spring force1/1
  M1P/1 -> MP/1
  connections:
  pin/RConn2 -- Custom Joint/LConn1
  Mechanical Branching Bar2/LConn1 -- Custom Joint/LConn2
  Mechanical Branching Bar1/LConn1 -- Custom Joint/RConn2
  L1D/LConn1 -- Link/RConn2
  L1U/LConn1 -- Link/LConn2
  pin/RConn1 -- M1P/LConn1
  M1P1/LConn1 -- pin/LConn1
  "Reaction Force Sensor "/LConn1 -- Mechanical Branching Bar1/RConn1
  Base/RConn1 -- pin/LConn2
  Follower/RConn1 -- Link/RConn1
  Custom Joint/RConn1 -- Link/LConn1
  Mechanical Branching Bar1/RConn2 -- Spring Lengh Sensor/LConn1
  Spring Contant/RConn1 -- Mechanical Branching Bar2/RConn1
  Spring Free Lenght/RConn1 -- Mechanical Branching Bar2/RConn2

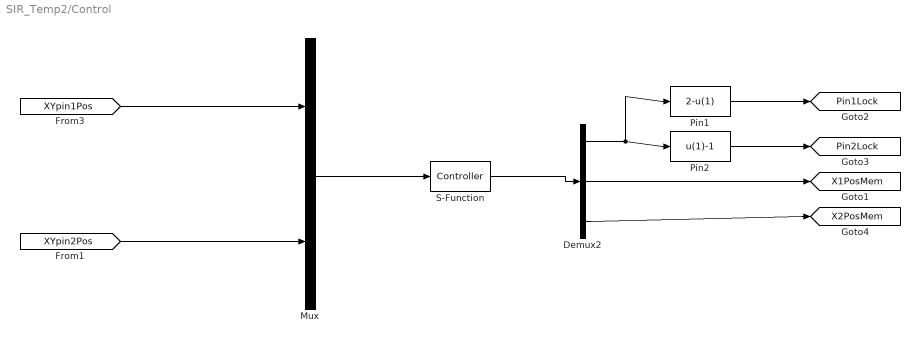
== system SIR_Temp2/Control ==
  Demux2 : Demux  Outputs=3
  Mux : Mux  Inputs=2
  Pin1 : Fcn  Expr=2-u(1)
  Pin2 : Fcn  Expr=u(1)-1
  S-Function : S-Function  FunctionName=Controller  Parameters=0.001  EnableBusSupport=off
  tag scope: Pin1Lock=global, Pin2Lock=global, X1PosMem=global, X2PosMem=global
  wires:
  Mux/1 -> S-Function/1
  Pin1/1 -> [Pin1Lock]
  Pin2/1 -> [Pin2Lock]
  [XYpin1Pos] -> Mux/1
  [XYpin2Pos] -> Mux/2
  S-Function/1 -> Demux2/1
  Demux2/1 -> Pin1/1, Pin2/1
  Demux2/2 -> [X1PosMem]
  Demux2/3 -> [X2PosMem]

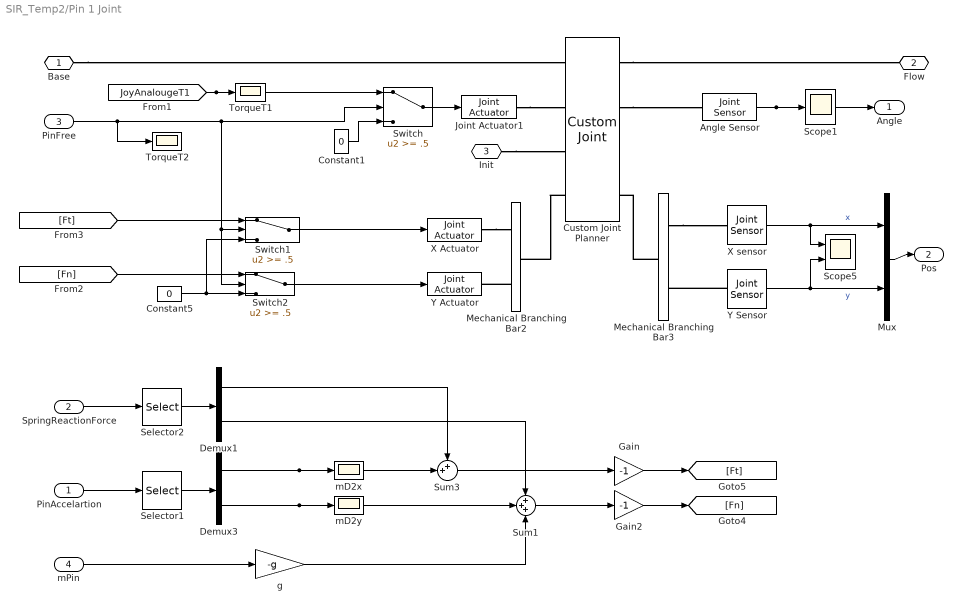
== system SIR_Temp2/Pin 1 Joint ==
  PinAccelartion : Inport
  SpringReactionForce : Inport  Port=2
  PinFree : Inport  Port=3
  mPin : Inport  Port=4
  Angle Sensor : mblibv1/Sensors &  Actuators/Joint Sensor  SystemSampleTime=-1  UpdateFromCAD=off  PhysicalDomain=Mechanical  PortType=blob  Muxed=off  Pose=off  Angle=on  AngleUnits=deg  ArcVelocity=off  ArcVelocityUnits=deg/s  ArcAcceleration=off  ArcAccelerationUnits=deg/s^2  CoordPosition=on  CoordPositionUnits=m  Velocity=off  VelocityUnits=m/s  Acceleration=off  AccelerationUnits=m/s^2  Quaternion=on  QuaternionDT=off  QuaternionDDT=off  QuaternionUnits=off  OutputVector=[1]  ActiveIO=on  Width=1  DialogClass=MechanicalSensorBlock  Primitive=R1  Force=off  ForceUnits=N  Torque=off  TorqueUnits=N*m  ReferenceFrame=Absolute (World)  ReactionSensedSide=Base  ReactionReferenceFrame=Absolute (World)  ReactionForce=off  ReactionForceUnits=N  ReactionMoment=off  ReactionMomentUnits=N*m
  Constant1 : Constant  Value=0
  Constant5 : Constant  Value=0
  Custom Joint Planner : mblibv1/Joints/Custom Joint  PhysicalDomain=mechanical  SubClassName=custom_joint  LeftPortType=blob  RightPortType=blob  LConnTagsString=__newl0|SA1|SA2|SA3  RConnTagsString=__newr0|SA1|SA2|SA3  UpdateFromCAD=off  NumSAPorts=6  CutJoint=off  MarkAsCut=off  Primitives=prismatic  PrimitiveProps="P1$World$[ 1 0  0]$Prismatic#P2$World$[0 1 0 ]$Prismatic#R1$World$[0 0 1]$Revolute"  DialogClass=JointBlock  R1Axis=[0 0 1]  R2Axis=[]  R3Axis=[]  P1Axis="[ 1 0  0]"  P2Axis=[0 1 0 ]  P3Axis=[]  SAxis=[]
  Demux1 : Demux  Outputs=2
  Demux3 : Demux  Outputs=2
  Gain : Gain  Gain=-1
  Gain2 : Gain  Gain=-1
  Joint Actuator1 : mblibv1/Sensors &  Actuators/Joint Actuator  SystemSampleTime=-1  UpdateFromCAD=off  PhysicalDomain=Mechanical  PortType=blob  ActuationStyle=Force  AngleUnits=deg  ArcVelocityUnits=deg/s  ArcAccelerationUnits=deg/s^2  CoordPositionUnits=m  VelocityUnits=m/s  AccelerationUnits=m/s^2  ForceUnits=N  TorqueUnits=N*m  ActiveIO=on  Width=1  DialogClass=MechanicalActuatorBlock  Primitive=R1  ReferenceFrame=Absolute (World)
  Mechanical Branching Bar2 : mblibv1/Utilities/Mechanical Branching Bar  PhysicalDomain=mechanical  SubClassName=Unknown  LeftPortType=blob  RightPortType=blob  LConnTagsString=_newl0  RConnTagsString=__newr0|SA2  UpdateFromCAD=off  DialogClass=MechanicalBranchingBarBlock  NumSAPorts=2
  Mechanical Branching Bar3 : mblibv1/Utilities/Mechanical Branching Bar  PhysicalDomain=mechanical  SubClassName=Unknown  LeftPortType=blob  RightPortType=blob  LConnTagsString=_newl0  RConnTagsString=__newr0|SA2  UpdateFromCAD=off  DialogClass=MechanicalBranchingBarBlock  NumSAPorts=2
  Mux : Mux  Inputs=2
  Scope1 : Scope
      settings: TimeRange=100  YMin=-1.25  YMax=1
  Scope5 : Scope  NumInputPorts=2
      settings: TimeRange=100  YMin=-1.25~0.65  YMax=1~1.025  SaveName=ScopeData9
  Selector1 : Selector  IndexMode=Zero-based  InputPortWidth=3  IndexOptions=Index vector (dialog)  Indices=[0 1]  OutputSizes=1
  Selector2 : Selector  IndexMode=Zero-based  InputPortWidth=3  IndexOptions=Index vector (dialog)  Indices=[0 1]  OutputSizes=1
  Sum1 : Sum  Inputs=+++
  Sum3 : Sum  Inputs=++|
  Switch : Switch  Threshold=.5
  Switch1 : Switch  Threshold=.5
  Switch2 : Switch  Threshold=.5
  TorqueT1 : Scope
      settings: TimeRange=100  YMin=-15  YMax=15
  TorqueT2 : Scope
      settings: TimeRange=100  YMin=-15  YMax=15  SaveName=ScopeData10
  "X Actuator " : mblibv1/Sensors &  Actuators/Joint Actuator  SystemSampleTime=-1  UpdateFromCAD=off  PhysicalDomain=Mechanical  PortType=blob  ActuationStyle=Force  AngleUnits=deg  ArcVelocityUnits=deg/s  ArcAccelerationUnits=deg/s^2  CoordPositionUnits=m  VelocityUnits=m/s  AccelerationUnits=m/s^2  ForceUnits=N  TorqueUnits=N*m  ActiveIO=on  Width=1  DialogClass=MechanicalActuatorBlock  Primitive=P1  ReferenceFrame=Absolute (World)
  X sensor : mblibv1/Sensors &  Actuators/Joint Sensor  SystemSampleTime=-1  UpdateFromCAD=off  PhysicalDomain=Mechanical  PortType=blob  Muxed=on  Pose=off  Angle=on  AngleUnits=deg  ArcVelocity=off  ArcVelocityUnits=deg/s  ArcAcceleration=off  ArcAccelerationUnits=deg/s^2  CoordPosition=on  CoordPositionUnits=m  Velocity=off  VelocityUnits=m/s  Acceleration=off  AccelerationUnits=m/s^2  Quaternion=on  QuaternionDT=off  QuaternionDDT=off  QuaternionUnits=off  OutputVector=[1]  ActiveIO=on  Width=1  DialogClass=MechanicalSensorBlock  Primitive=P1  Force=off  ForceUnits=N  Torque=off  TorqueUnits=N*m  ReferenceFrame=Absolute (World)  ReactionSensedSide=Follower  ReactionReferenceFrame=Absolute (World)  ReactionForce=off  ReactionForceUnits=N  ReactionMoment=off  ReactionMomentUnits=N*m
  Y Actuator : mblibv1/Sensors &  Actuators/Joint Actuator  SystemSampleTime=-1  UpdateFromCAD=off  PhysicalDomain=Mechanical  PortType=blob  ActuationStyle=Force  AngleUnits=deg  ArcVelocityUnits=deg/s  ArcAccelerationUnits=deg/s^2  CoordPositionUnits=m  VelocityUnits=m/s  AccelerationUnits=m/s^2  ForceUnits=N  TorqueUnits=N*m  ActiveIO=on  Width=1  DialogClass=MechanicalActuatorBlock  Primitive=P2  ReferenceFrame=Absolute (World)
  Y Sensor : mblibv1/Sensors &  Actuators/Joint Sensor  SystemSampleTime=-1  UpdateFromCAD=off  PhysicalDomain=Mechanical  PortType=blob  Muxed=on  Pose=off  Angle=on  AngleUnits=deg  ArcVelocity=off  ArcVelocityUnits=deg/s  ArcAcceleration=off  ArcAccelerationUnits=deg/s^2  CoordPosition=on  CoordPositionUnits=m  Velocity=off  VelocityUnits=m/s  Acceleration=off  AccelerationUnits=m/s^2  Quaternion=on  QuaternionDT=off  QuaternionDDT=off  QuaternionUnits=off  OutputVector=[1]  ActiveIO=on  Width=1  DialogClass=MechanicalSensorBlock  Primitive=P2  Force=off  ForceUnits=N  Torque=off  TorqueUnits=N*m  ReferenceFrame=Absolute (World)  ReactionSensedSide=Follower  ReactionReferenceFrame=Absolute (World)  ReactionForce=off  ReactionForceUnits=N  ReactionMoment=off  ReactionMomentUnits=N*m
  g : Gain  Gain=-g
  mD2x : Scope
      settings: TimeRange=100  YMin=-3.5  YMax=4.5  SaveName=ScopeData14
  mD2y : Scope
      settings: TimeRange=1.4  YMin=-9e-16  YMax=1.4e-15  SaveName=ScopeData15
  Base : PMIOPort  Port=1  Side=Left
  Flow : PMIOPort  Port=2  Side=Right
  Init : PMIOPort  Port=3  Side=Left
  Angle : Outport
  Pos : Outport  Port=2
  wires:
  PinFree/1 -> TorqueT2/1, Switch/2, Switch1/2, Switch2/2
  Y Sensor/1 -> Scope5/2, Mux/2  "y"
  X sensor/1 -> Scope5/1, Mux/1  "x"
  [JoyAnalougeT1] -> Switch/1, TorqueT1/1
  Angle Sensor/1 -> Scope1/1, Angle/1
  Switch/1 -> Joint Actuator1/1
  Constant1/1 -> Switch/3
  Constant5/1 -> Switch1/3, Switch2/3
  [Fn] -> Switch2/1
  [Ft] -> Switch1/1
  mPin/1 -> g/1
  Demux3/1 -> Sum3/2, mD2x/1
  Demux3/2 -> Sum1/2, mD2y/1
  Sum1/1 -> Gain2/1
  Gain2/1 -> [Fn]
  Sum3/1 -> Gain/1
  Gain/1 -> [Ft]
  PinAccelartion/1 -> Selector1/1
  Selector1/1 -> Demux3/1
  g/1 -> Sum1/3
  Selector2/1 -> Demux1/1
  SpringReactionForce/1 -> Selector2/1
  Demux1/1 -> Sum3/1
  Demux1/2 -> Sum1/1
  Mux/1 -> Pos/1
  Switch1/1 -> "X Actuator "/1
  Switch2/1 -> Y Actuator/1
  connections:
  "X Actuator "/RConn1 -- Mechanical Branching Bar2/RConn1
  Y Sensor/LConn1 -- Mechanical Branching Bar3/RConn2
  Mechanical Branching Bar3/RConn1 -- X sensor/LConn1
  Mechanical Branching Bar2/RConn2 -- Y Actuator/RConn1
  Mechanical Branching Bar3/LConn1 -- Custom Joint Planner/RConn4
  Custom Joint Planner/LConn4 -- Mechanical Branching Bar2/LConn1
  Init/RConn1 -- Custom Joint Planner/LConn3
  Joint Actuator1/RConn1 -- Custom Joint Planner/LConn2
  Custom Joint Planner/RConn2 -- Angle Sensor/LConn1
  Custom Joint Planner/RConn1 -- Flow/RConn1
  Base/RConn1 -- Custom Joint Planner/LConn1

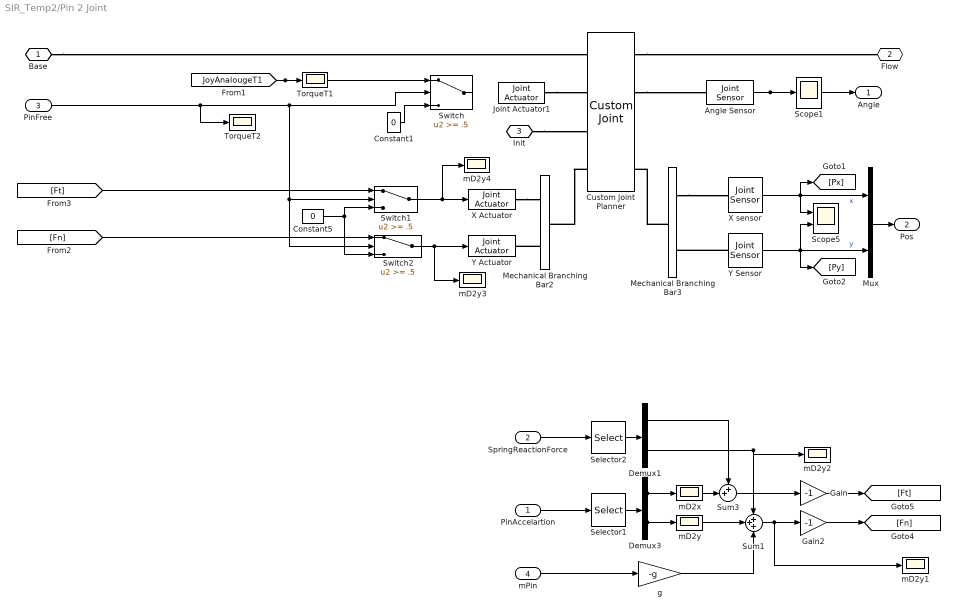
== system SIR_Temp2/Pin 2 Joint ==
  PinAccelartion : Inport
  SpringReactionForce : Inport  Port=2
  PinFree : Inport  Port=3
  mPin : Inport  Port=4
  Angle Sensor : mblibv1/Sensors &  Actuators/Joint Sensor  SystemSampleTime=-1  UpdateFromCAD=off  PhysicalDomain=Mechanical  PortType=blob  Muxed=off  Pose=off  Angle=on  AngleUnits=deg  ArcVelocity=off  ArcVelocityUnits=deg/s  ArcAcceleration=off  ArcAccelerationUnits=deg/s^2  CoordPosition=on  CoordPositionUnits=m  Velocity=off  VelocityUnits=m/s  Acceleration=off  AccelerationUnits=m/s^2  Quaternion=on  QuaternionDT=off  QuaternionDDT=off  QuaternionUnits=off  OutputVector=[1]  ActiveIO=on  Width=1  DialogClass=MechanicalSensorBlock  Primitive=R1  Force=off  ForceUnits=N  Torque=off  TorqueUnits=N*m  ReferenceFrame=Absolute (World)  ReactionSensedSide=Base  ReactionReferenceFrame=Absolute (World)  ReactionForce=off  ReactionForceUnits=N  ReactionMoment=off  ReactionMomentUnits=N*m
  Constant1 : Constant  Value=0
  Constant5 : Constant  Value=0
  Custom Joint Planner : mblibv1/Joints/Custom Joint  PhysicalDomain=mechanical  SubClassName=custom_joint  LeftPortType=blob  RightPortType=blob  LConnTagsString=__newl0|SA1|SA2|SA3  RConnTagsString=__newr0|SA1|SA2|SA3  UpdateFromCAD=off  NumSAPorts=6  CutJoint=off  MarkAsCut=off  Primitives=prismatic  PrimitiveProps="P1$World$[ 1 0  0]$Prismatic#P2$World$[0 1 0 ]$Prismatic#R1$World$[0 0 1]$Revolute"  DialogClass=JointBlock  R1Axis=[0 0 1]  R2Axis=[]  R3Axis=[]  P1Axis="[ 1 0  0]"  P2Axis=[0 1 0 ]  P3Axis=[]  SAxis=[]
  Demux1 : Demux  Outputs=2
  Demux3 : Demux  Outputs=2
  Gain : Gain  Gain=-1
  Gain2 : Gain  Gain=-1
  Joint Actuator1 : mblibv1/Sensors &  Actuators/Joint Actuator  SystemSampleTime=-1  UpdateFromCAD=off  PhysicalDomain=Mechanical  PortType=blob  ActuationStyle=Force  AngleUnits=deg  ArcVelocityUnits=deg/s  ArcAccelerationUnits=deg/s^2  CoordPositionUnits=m  VelocityUnits=m/s  AccelerationUnits=m/s^2  ForceUnits=N  TorqueUnits=N*m  ActiveIO=on  Width=1  DialogClass=MechanicalActuatorBlock  Primitive=R1  ReferenceFrame=Absolute (World)
  Mechanical Branching Bar2 : mblibv1/Utilities/Mechanical Branching Bar  PhysicalDomain=mechanical  SubClassName=Unknown  LeftPortType=blob  RightPortType=blob  LConnTagsString=_newl0  RConnTagsString=__newr0|SA2  UpdateFromCAD=off  DialogClass=MechanicalBranchingBarBlock  NumSAPorts=2
  Mechanical Branching Bar3 : mblibv1/Utilities/Mechanical Branching Bar  PhysicalDomain=mechanical  SubClassName=Unknown  LeftPortType=blob  RightPortType=blob  LConnTagsString=_newl0  RConnTagsString=__newr0|SA2  UpdateFromCAD=off  DialogClass=MechanicalBranchingBarBlock  NumSAPorts=2
  Mux : Mux  Inputs=2
  Scope1 : Scope
      settings: TimeRange=100  YMin=-1.25  YMax=1
  Scope5 : Scope  NumInputPorts=2
      settings: TimeRange=100  YMin=-1.25~0.65  YMax=1~1.025  SaveName=ScopeData9
  Selector1 : Selector  IndexMode=Zero-based  InputPortWidth=3  IndexOptions=Index vector (dialog)  Indices=[0 1]  OutputSizes=1
  Selector2 : Selector  IndexMode=Zero-based  InputPortWidth=3  IndexOptions=Index vector (dialog)  Indices=[0 1]  OutputSizes=1
  Sum1 : Sum  Inputs=+++
  Sum3 : Sum  Inputs=++|
  Switch : Switch  Threshold=.5
  Switch1 : Switch  Threshold=.5
  Switch2 : Switch  Threshold=.5
  TorqueT1 : Scope
      settings: TimeRange=100  YMin=-15  YMax=15
  TorqueT2 : Scope
      settings: TimeRange=100  YMin=-15  YMax=15  SaveName=ScopeData10
  "X Actuator " : mblibv1/Sensors &  Actuators/Joint Actuator  SystemSampleTime=-1  UpdateFromCAD=off  PhysicalDomain=Mechanical  PortType=blob  ActuationStyle=Force  AngleUnits=deg  ArcVelocityUnits=deg/s  ArcAccelerationUnits=deg/s^2  CoordPositionUnits=m  VelocityUnits=m/s  AccelerationUnits=m/s^2  ForceUnits=N  TorqueUnits=N*m  ActiveIO=on  Width=1  DialogClass=MechanicalActuatorBlock  Primitive=P1  ReferenceFrame=Absolute (World)
  X sensor : mblibv1/Sensors &  Actuators/Joint Sensor  SystemSampleTime=-1  UpdateFromCAD=off  PhysicalDomain=Mechanical  PortType=blob  Muxed=on  Pose=off  Angle=on  AngleUnits=deg  ArcVelocity=off  ArcVelocityUnits=deg/s  ArcAcceleration=off  ArcAccelerationUnits=deg/s^2  CoordPosition=on  CoordPositionUnits=m  Velocity=off  VelocityUnits=m/s  Acceleration=off  AccelerationUnits=m/s^2  Quaternion=on  QuaternionDT=off  QuaternionDDT=off  QuaternionUnits=off  OutputVector=[1]  ActiveIO=on  Width=1  DialogClass=MechanicalSensorBlock  Primitive=P1  Force=off  ForceUnits=N  Torque=off  TorqueUnits=N*m  ReferenceFrame=Absolute (World)  ReactionSensedSide=Follower  ReactionReferenceFrame=Absolute (World)  ReactionForce=off  ReactionForceUnits=N  ReactionMoment=off  ReactionMomentUnits=N*m
  Y Actuator : mblibv1/Sensors &  Actuators/Joint Actuator  SystemSampleTime=-1  UpdateFromCAD=off  PhysicalDomain=Mechanical  PortType=blob  ActuationStyle=Force  AngleUnits=deg  ArcVelocityUnits=deg/s  ArcAccelerationUnits=deg/s^2  CoordPositionUnits=m  VelocityUnits=m/s  AccelerationUnits=m/s^2  ForceUnits=N  TorqueUnits=N*m  ActiveIO=on  Width=1  DialogClass=MechanicalActuatorBlock  Primitive=P2  ReferenceFrame=Absolute (World)
  Y Sensor : mblibv1/Sensors &  Actuators/Joint Sensor  SystemSampleTime=-1  UpdateFromCAD=off  PhysicalDomain=Mechanical  PortType=blob  Muxed=on  Pose=off  Angle=on  AngleUnits=deg  ArcVelocity=off  ArcVelocityUnits=deg/s  ArcAcceleration=off  ArcAccelerationUnits=deg/s^2  CoordPosition=on  CoordPositionUnits=m  Velocity=off  VelocityUnits=m/s  Acceleration=off  AccelerationUnits=m/s^2  Quaternion=on  QuaternionDT=off  QuaternionDDT=off  QuaternionUnits=off  OutputVector=[1]  ActiveIO=on  Width=1  DialogClass=MechanicalSensorBlock  Primitive=P2  Force=off  ForceUnits=N  Torque=off  TorqueUnits=N*m  ReferenceFrame=Absolute (World)  ReactionSensedSide=Follower  ReactionReferenceFrame=Absolute (World)  ReactionForce=off  ReactionForceUnits=N  ReactionMoment=off  ReactionMomentUnits=N*m
  g : Gain  Gain=-g
  mD2x : Scope
      settings: TimeRange=100  YMin=-3.5  YMax=4.5  SaveName=ScopeData14
  mD2y{,1..4} (5 alike) : Scope
      mD2y settings: TimeRange=1.4  YMin=-9e-16  YMax=1.4e-15  SaveName=ScopeData15
      mD2y1 settings: TimeRange=0.7000000000000001  YMin=-10  YMax=25  SaveName=ScopeData2
      mD2y2 settings: TimeRange=0.7000000000000001  YMin=-10  YMax=30  SaveName=ScopeData3
      mD2y3 settings: TimeRange=0.7000000000000001  YMin=-10  YMax=30  SaveName=ScopeData4
      mD2y4 settings: TimeRange=0.7000000000000001  YMin=-10  YMax=30  SaveName=ScopeData5
  Base : PMIOPort  Port=1  Side=Left
  Flow : PMIOPort  Port=2  Side=Right
  Init : PMIOPort  Port=3  Side=Left
  Angle : Outport
  Pos : Outport  Port=2
  wires:
  PinFree/1 -> TorqueT2/1, Switch/2, Switch1/2, Switch2/2
  Y Sensor/1 -> Scope5/2, Mux/2, [Py]  "y"
  X sensor/1 -> Scope5/1, Mux/1, [Px]  "x"
  [JoyAnalougeT1] -> Switch/1, TorqueT1/1
  Angle Sensor/1 -> Scope1/1, Angle/1
  Constant1/1 -> Switch/3
  mPin/1 -> g/1
  Demux3/1 -> Sum3/2, mD2x/1
  Demux3/2 -> mD2y/1, Sum1/2
  Sum1/1 -> Gain2/1, mD2y1/1
  Gain2/1 -> [Fn]
  Sum3/1 -> Gain/1
  Gain/1 -> [Ft]
  PinAccelartion/1 -> Selector1/1
  Selector1/1 -> Demux3/1
  g/1 -> Sum1/3
  Selector2/1 -> Demux1/1
  SpringReactionForce/1 -> Selector2/1
  Demux1/1 -> Sum3/1
  Demux1/2 -> Sum1/1, mD2y2/1
  Mux/1 -> Pos/1
  Switch1/1 -> "X Actuator "/1, mD2y4/1
  Switch2/1 -> Y Actuator/1, mD2y3/1
  [Fn] -> Switch2/1
  Constant5/1 -> Switch1/3, Switch2/3
  [Ft] -> Switch1/1
  connections:
  "X Actuator "/RConn1 -- Mechanical Branching Bar2/RConn1
  Y Sensor/LConn1 -- Mechanical Branching Bar3/RConn2
  Mechanical Branching Bar3/RConn1 -- X sensor/LConn1
  Mechanical Branching Bar2/RConn2 -- Y Actuator/RConn1
  Mechanical Branching Bar3/LConn1 -- Custom Joint Planner/RConn4
  Custom Joint Planner/LConn4 -- Mechanical Branching Bar2/LConn1
  Init/RConn1 -- Custom Joint Planner/LConn3
  Joint Actuator1/RConn1 -- Custom Joint Planner/LConn2
  Custom Joint Planner/RConn2 -- Angle Sensor/LConn1
  Custom Joint Planner/RConn1 -- Flow/RConn1
  Base/RConn1 -- Custom Joint Planner/LConn1
